simulink model "surge_model_controlled"  (R2014a)
settings: Solver=ode45  StartTime=tstart  StopTime=tstop  RelTol=1e-3
values from neighbouring files (symbols this model uses):
  T = 500    [run_task_1_7.m]
settings Model: Creator=Hwk  LastModifiedBy=Hwk

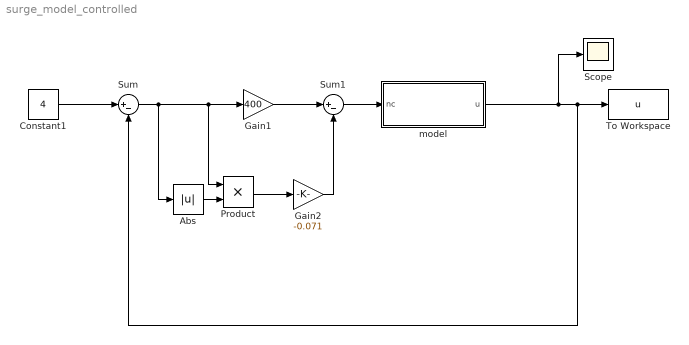
== system surge_model_controlled ==
  Abs : Abs
  Constant1 : Constant  Value=4
  Gain1 : Gain  Gain=400
  Gain2 : Gain  Gain=-0.071
  Product : Product
  Scope : Scope
  Sum : Sum  Inputs=|+-
  Sum1 : Sum  Inputs=|+-
  To Workspace : ToWorkspace  VariableName=u  SampleTime=10
  model : Subsystem
  wires:
  model/1(u) -> Scope/1, Sum/2, To Workspace/1
  Constant1/1 -> Sum/1
  Product/1 -> Gain2/1
  Gain2/1 -> Sum1/2
  Sum/1 -> Abs/1, Gain1/1, Product/1
  Abs/1 -> Product/2
  Sum1/1 -> model/1(nc)
  Gain1/1 -> Sum1/1

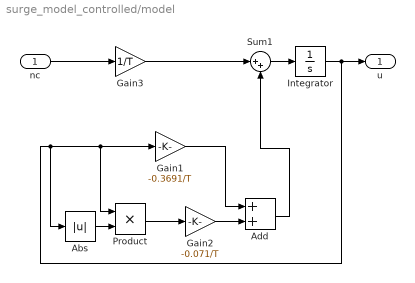
== system surge_model_controlled/model ==
  nc : Inport
  Abs : Abs
  Add : Sum
  Gain1 : Gain  Gain=-0.3691/T
  Gain2 : Gain  Gain=-0.071/T
  Gain3 : Gain  Gain=1/T
  Integrator : Integrator
  Product : Product
  Sum1 : Sum  Inputs=|++
  u : Outport
  wires:
  nc/1 -> Gain3/1
  Gain3/1 -> Sum1/1
  Gain1/1 -> Add/1
  Sum1/1 -> Integrator/1
  Product/1 -> Gain2/1
  Gain2/1 -> Add/2
  Add/1 -> Sum1/2
  Integrator/1 -> Gain1/1, Product/1, Abs/1, u/1
  Abs/1 -> Product/2
